simulink model "WEankle_controllerMaarten_2018"  (R2018b)
settings: Solver=FixedStepDiscrete  StartTime=0.0  StopTime=inf  FixedStep=sampleTime  RelTol=1e-3
PreLoadFcn:
  | init
undefined symbols (not defined in the file or in its folder): DiscIntNeverNeededParam, forceplate, Joint_params, sampleTime
libraries: simulink x21, WE2_library x9, dspsigops x6, dspfdesign x3
(part 2 of 4)

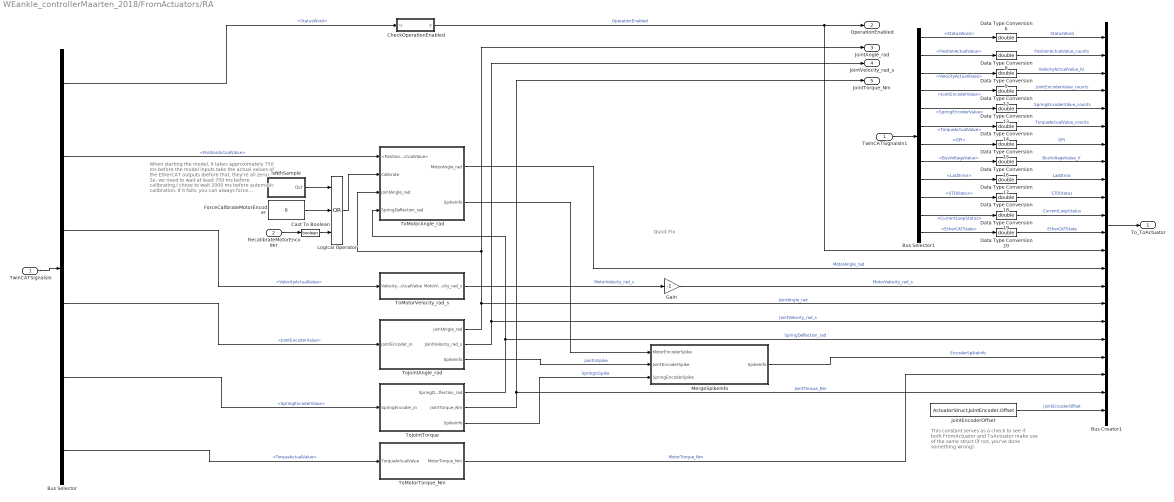
== system WEankle_controllerMaarten_2018/FromActuators/RA ==
  note: Quick Fix
  note: When starting the model, it takes approximately 750 ms before the model inputs take the actual values of the EtherCAT outputs (before that, they're all zero). So, we need to wait at least 750 ms before calibrating.I chose to wait 2000 ms before automatic calibration.
      |
      | If it fails, you can always force re-calibration.
  note: This constant serves as a check to see if both FromActuator and ToActuator make use of the same struct (if not, you've done something wrong).
  TwinCATSignalsIn : Inport  OutDataTypeStr=Bus: WE_InputBus
  RecalibrateMotorEncoder : Inport  Port=2
  Bus Creator1 : BusCreator  Inputs=22  OutDataTypeStr=Bus: WE_ToToActuatorBus  NonVirtualBus=on
      settings: InheritFromInputs=off
  Bus Selector : BusSelector  OutputSignals=StatusWord,PositionActualValue,VelocityActualValue,JointEncoderValue,SpringEncoderValue,TorqueActualValue
  Bus Selector1 : BusSelector  OutputSignals=StatusWord,PositionActualValue,VelocityActualValue,JointEncoderValue,SpringEncoderValue,TorqueActualValue,GPI,BusVoltageValue,LastError,STOStatus,CurrentLoopStatus,EtherCATState
  Cast To Boolean : DataTypeConversion  OutDataTypeStr=boolean
  CheckOperationEnabled : MATLAB Function  TreatAsAtomicUnit=on
  Data Type Conversion{6,8..9,12..20} (12 alike) : DataTypeConversion  OutDataTypeStr=double
  ForceCalibrateMotorEncoder : Constant  Value=0
      settings: OpenFcn=set_param(gcb,'Value','1');tname = ['toggletimer_' gcb];delete(timerfind('name',tname));t = timer('timerfcn', ['set_param(''',gcb,''',''Value'',''0'')'],'executionmode','singleshot','startdelay',1,'name',tname);start(t);
      mask Display: fprintf('PushToTrigger\n%s',get_param(gcb,'value'))
  Gain : Gain  Gain=-1
  IsNthSample : Subsystem  InitFcn=|  mask{N=2000}
      | return; %Disable this becasue it doesnt work!                                                                                                                                                          
      | h = gcb;                                                                                                                                                                                               
      | n = 0; % Number of enable blocks detected upstream                                                                                                                                                     
      | t = []; % type of enable blocks                                                                                                                                                                        
      | while 1,                                                                                                                                                                                               
      |   % Find parent                                                                                                                                                                                        
      |   h = get_param(h,'parent');                                                                                                                                                                           
      |   if (strcmp(h,'')),                                                                                                                                                                                   
      |       % Then we've reached the root                                                                                                                                                                    
      |       break;                                                                                                                                                                                           
      |   end;                                                                                                                                                                                                 
      |   % and check if it has an enable port                                                                                                                                                                 
      |   e = find_system(h,'searchdepth',1, 'BlockType','EnablePort');                                                                                                                                        
      |   if (numel(e)==1),                                                                                                                                                                                    
      |     s = get_param(e{1},'StatesWhenEnabling');                                                                                                                                                          
      |     n=n+1;                                                                                                                                                                                             
      |     if (strcmp(s,'held')),                                                                                                                                                                             
      |         t=[t;'h']; %#ok<AGROW>                                                                                                                                                                         
      |     else                                                                                                                                                                                               
      |         t=[t;'r']; %#ok<AGROW>                                                                                                                                                                         
      |     end;                                                                                                                                                                                               
      |   elseif (numel(e)>1),                                                                                                                                                                                 
      |       error('hun? Multiple enable blocks!')                                                                                                                                                            
      |   end;                                                                                                                                                                                                 
      | end;                                                                                                                                                                                                   
      |                                                                                                                                                                                                        
      | if (n==0),                                                                                                                                                                                             
      |     warning('Warning: %s - The block is not inside an enabled block',gcb)                                                                                                                              
      | elseif (n==1),                                                                                                                                                                                         
      |     if (t(1)=='r')                                                                                                                                                                                     
      |         % This is okay, do nothing                                                                                                                                                                     
      |     else                                                                                                                                                                                               
      |         warning('Warning: %s - This block is inside an enabled block which has its "State when enabling" set to "held". Usually you want it set to "reset" for correct operation.',gcb);               
      |     end;                                                                                                                                                                                               
      | else % n>1                                                                                                                                                                                             
      |     warning('Warning: %s - This block is inside multiple nested enabled blocks. Check which blocks are "held" and which are "reset". You usually want to have at least one "reset" enabled block',gcb);
      | end;
  JointEncoderOffset : Constant  Value=ActuatorStruct.JointEncoder.Offset
  Logical Operator : Logic  Operator=OR  Inputs=3  AllPortsSameDT=off  OutDataTypeStr=boolean
  MergeSpikeInfo : Subsystem
  ToJointAngle_rad : Subsystem
  ToJointTorque : Subsystem
  ToMotorAngle_rad : Subsystem
  ToMotorTorque_Nm : Subsystem
  ToMotorVelocity_rad_s : Subsystem
  TwinCATSignalsIn1 : InportShadow  OutDataTypeStr=Bus: WE_InputBus
  To_ToActuator : Outport  OutDataTypeStr=Bus: WE_ToToActuatorBus  VectorParamsAs1DForOutWhenUnconnected=off
  OperationEnabled : Outport  Port=2  VectorParamsAs1DForOutWhenUnconnected=off
  JointAngle_rad : Outport  Port=3  VectorParamsAs1DForOutWhenUnconnected=off
  JointVelocity_rad_s : Outport  Port=4  VectorParamsAs1DForOutWhenUnconnected=off
  JointTorque_Nm : Outport  Port=5  VectorParamsAs1DForOutWhenUnconnected=off
  wires:
  Cast To Boolean/1 -> Logical Operator/3
  ToMotorAngle_rad/1(MotorAngle_rad) -> Bus Creator1/14  "MotorAngle_rad"
  Logical Operator/1 -> ToMotorAngle_rad/2(Calibrate)
  Bus Selector/2 -> ToMotorAngle_rad/1(<PositionActualValue>)  "<PositionActualValue>"
  ToMotorAngle_rad/2(SpikeInfo) -> MergeSpikeInfo/1(MotorEncoderSpike)
  MergeSpikeInfo/1(SpikeInfo) -> Bus Creator1/19  "EncoderSpikeInfo"
  Bus Selector1/12 -> Data Type Conversion20/1  "<EtherCATState>"
  Bus Selector1/11 -> Data Type Conversion19/1  "<CurrentLoopStatus>"
  Bus Selector1/10 -> Data Type Conversion18/1  "<STOStatus>"
  Bus Selector1/9 -> Data Type Conversion17/1  "<LastError>"
  Bus Selector1/8 -> Data Type Conversion16/1  "<BusVoltageValue>"
  Bus Selector1/7 -> Data Type Conversion15/1  "<GPI>"
  Bus Selector1/6 -> Data Type Conversion14/1  "<TorqueActualValue>"
  Bus Selector1/5 -> Data Type Conversion13/1  "<SpringEncoderValue>"
  Bus Selector1/4 -> Data Type Conversion12/1  "<JointEncoderValue>"
  Bus Selector1/3 -> Data Type Conversion9/1  "<VelocityActualValue>"
  Bus Selector1/2 -> Data Type Conversion8/1  "<PositionActualValue>"
  Data Type Conversion20/1 -> Bus Creator1/12  "EtherCATState"
  Data Type Conversion19/1 -> Bus Creator1/11  "CurrentLoopStatus"
  Data Type Conversion18/1 -> Bus Creator1/10  "STOStatus"
  Data Type Conversion17/1 -> Bus Creator1/9  "LastError"
  Data Type Conversion16/1 -> Bus Creator1/8  "BusVoltageValue_V"
  Data Type Conversion15/1 -> Bus Creator1/7  "GPI"
  Data Type Conversion14/1 -> Bus Creator1/6  "TorqueActualValue_counts"
  Data Type Conversion13/1 -> Bus Creator1/5  "SpringEncoderValue_counts"
  Data Type Conversion12/1 -> Bus Creator1/4  "JointEncoderValue_counts"
  Data Type Conversion9/1 -> Bus Creator1/3  "VelocityActualValue_IU"
  Data Type Conversion8/1 -> Bus Creator1/2  "PositionActualValue_counts"
  Data Type Conversion6/1 -> Bus Creator1/1  "StatusWord"
  Bus Selector1/1 -> Data Type Conversion6/1  "<StatusWord>"
  TwinCATSignalsIn1/1 -> Bus Selector1/1
  Bus Selector/6 -> ToMotorTorque_Nm/1(TorqueActualValue)  "<TorqueActualValue>"
  Bus Selector/5 -> ToJointTorque/1(SpringEncoder_in)  "<SpringEncoderValue>"
  Bus Selector/4 -> ToJointAngle_rad/1(JointEncoder_in)  "<JointEncoderValue>"
  RecalibrateMotorEncoder/1 -> Cast To Boolean/1
  ToMotorVelocity_rad_s/1(MotorVelocity_rad_s) -> Gain/1  "MotorVelocity_rad_s"
  ToMotorTorque_Nm/1(MotorTorque_Nm) -> Bus Creator1/20  "MotorTorque_Nm"
  ToJointTorque/3(SpikeInfo) -> MergeSpikeInfo/3(SpringEncoderSpike)  "SpringIsSpike"
  ToJointAngle_rad/3(SpikeInfo) -> MergeSpikeInfo/2(JointEncoderSpike)  "JointIsSpike"
  JointEncoderOffset/1 -> Bus Creator1/22  "JointEncoderOffset"
  Bus Creator1/1 -> To_ToActuator/1
  CheckOperationEnabled/1(y) -> OperationEnabled/1, Bus Creator1/13  "OperationEnabled"
  ToJointTorque/2(JointTorque_Nm) -> Bus Creator1/21, JointTorque_Nm/1  "JointTorque_Nm"
  ToJointAngle_rad/2(JointVelocity_rad_s) -> Bus Creator1/17, JointVelocity_rad_s/1  "JointVelocity_rad_s"
  ToJointAngle_rad/1(JointAngle_rad) -> ToMotorAngle_rad/3(JointAngle_rad), JointAngle_rad/1, Bus Creator1/16  "JointAngle_rad"
  ToJointTorque/1(SpringDeflection_rad) -> ToMotorAngle_rad/4(SpringDeflection_rad), Bus Creator1/18  "SpringDeflection_rad"
  IsNthSample/1(Out) -> Logical Operator/1
  ForceCalibrateMotorEncoder/1 -> Logical Operator/2
  TwinCATSignalsIn/1 -> Bus Selector/1
  Bus Selector/1 -> CheckOperationEnabled/1(u)  "<StatusWord>"
  Bus Selector/3 -> ToMotorVelocity_rad_s/1(VelocityActualValue)  "<VelocityActualValue>"
  Gain/1 -> Bus Creator1/15  "MotorVelocity_rad_s"

== system WEankle_controllerMaarten_2018/Ankle Controller/COMverror and perturbation/COMvError ==
  note: This input signal should be taken from original, but the data is not good before the filter because of the Qualisys sample rate
  Signaltime : Inport
  trigger : Inport  Port=2
  xPosCOM : Inport  Port=3
  Constant : Constant  Value=5
  Constant1 : Constant  Value=1.5
  Data lost detection : Subsystem
  MATLAB Function1 : MATLAB Function  TreatAsAtomicUnit=on
  PertDetection : Subsystem
  PerturbationDetectionFromError : MATLAB Function  TreatAsAtomicUnit=on
  Signal learner : Subsystem
  Terminator : Terminator
  Terminator1 : Terminator
  Terminator8 : Terminator
  to mm : Gain  Gain=1000
  PushDetected : Outport  VectorParamsAs1DForOutWhenUnconnected=off
  COMv_meas : Outport  Port=2  VectorParamsAs1DForOutWhenUnconnected=off
  COMv_ref : Outport  Port=3  VectorParamsAs1DForOutWhenUnconnected=off
  COMv_error : Outport  Port=4  VectorParamsAs1DForOutWhenUnconnected=off
  tag scope: DataLost=global, ShutDown=global
  wires:
  to mm/1 -> Signal learner/3(xPosCOM)
  [ShutDown] -> MATLAB Function1/1(ShutDown)
  PertDetection/1(PertDetect) -> MATLAB Function1/2(PertDetect)
  Signal learner/6(ShutDown) -> [ShutDown]
  [DataLost] -> PerturbationDetectionFromError/6(DataLost)
  Data lost detection/2(DataLost) -> [DataLost]  "DataLost"
  Constant1/1 -> PerturbationDetectionFromError/5(threshPert)
  Signal learner/3(Input filtered) -> Data lost detection/1(Input signal), COMv_meas/1  "InputFiltered"
  Data lost detection/1(New error) -> COMv_error/1, PerturbationDetectionFromError/3(signal)  "Error"
  Signal learner/4(learned) -> COMv_ref/1  "SignalLearned"
  MATLAB Function1/1(TriggerPush) -> PushDetected/1
  Data lost detection/3(avoid) -> PertDetection/3(avoid)
  Signal learner/5(Perturbation detected FromInput) -> PertDetection/2(PertFromInputSignal)
  PerturbationDetectionFromError/1(push) -> PertDetection/1(PertFromError)  "PertFromError"
  Constant/1 -> PerturbationDetectionFromError/4(n_rep)
  Signal learner/2(error) -> Data lost detection/2(ErrorIn)
  xPosCOM/1 -> to mm/1
  Signaltime/1 -> PerturbationDetectionFromError/1(t), Signal learner/1(Signaltime)
  trigger/1 -> Signal learner/2(trigger), PerturbationDetectionFromError/2(trigger)  "trigger"
  PerturbationDetectionFromError/2(maxAver) -> Terminator8/1
  PerturbationDetectionFromError/3(rangeAver) -> Terminator1/1
  Signal learner/1(original) -> Terminator/1

== system WEankle_controllerMaarten_2018/Ankle Controller/COMverror and perturbation/TriggerPerturbation ==
  note: Put it in 4
  note: I have to try the pull perturbation in the pusher and its response
      | and change the amplitude based on that
  note: 1 - only push
      | 0 - push and pull
  In1 : Inport
  In2 : Inport  Port=2
  SingleR : Inport  Port=3
  SingleL : Inport  Port=4
  In5 : Inport  Port=5
  In6 : Inport  Port=6
  Delay : Delay  DelayLength=200
  Demux2 : Demux  Outputs=2
  GainP : Gain  Gain=4
  MATLAB Function2 : MATLAB Function  TreatAsAtomicUnit=on
  Multiply1 : Product
  Perturbation sync gait phase1 : Subsystem
  PushOrPull : MATLAB Function  TreatAsAtomicUnit=on
  Selector4 : Selector  InputPortWidth=6  IndexOptions=Index vector (dialog)  Indices=3  OutputSizes=1
  Switch2 : Switch  Criteria=u2 > Threshold
  Terminator1 : Terminator
  Type of perturbations (random) : Constant  Value=[1 1 1 1 1 1 1 1 1]
  VectorOnlyPush : Constant
  VectorPushPull : Constant  Value=[1 -1 1 1 1 -1 -1 1 -1 -1 1 -1]
  PerturbationTrigger : Outport
  wires:
  In2/1 -> Switch2/2
  In1/1 -> Multiply1/1
  SingleR/1 -> MATLAB Function2/1(SingleR)
  In5/1 -> Demux2/1
  SingleL/1 -> MATLAB Function2/2(SingleL)
  Delay/1 -> PushOrPull/3(Delivered)
  PushOrPull/1(NewPert) -> GainP/1  "New pert"
  Perturbation sync gait phase1/3(allow) -> Terminator1/1
  Selector4/1 -> MATLAB Function2/5(GRFzL)
  VectorOnlyPush/1 -> Switch2/1
  Type of perturbations (random)/1 -> MATLAB Function2/6(TypePert)
  MATLAB Function2/1(Trigger) -> Perturbation sync gait phase1/1(trigger)  "trigger"
  Switch2/1 -> PushOrPull/2(vectorPushPull)  "vectorPert"
  Demux2/1 -> MATLAB Function2/3(PhaseL)  "PhaseL"
  VectorPushPull/1 -> Switch2/3
  In6/1 -> Selector4/1
  Demux2/2 -> MATLAB Function2/4(PhaseR)  "PhaseR"
  GainP/1 -> Multiply1/2
  Perturbation sync gait phase1/1(Pert sync) -> PushOrPull/1(Perturb)  "pert"
  Multiply1/1 -> PerturbationTrigger/1
  Perturbation sync gait phase1/2(Delivered) -> MATLAB Function2/7(Delivered), Delay/1  "Delivered"

== system WEankle_controllerMaarten_2018/Ankle Controller/Gait Phase detection/COP detection (treadmill) ==
  note: Detection of ground contact when wearing exo 200 (without exo 80)
  note: Number coding :
      | 1 = LIFOR
      | 2 = SSL
      | 3 = RIFOL
      | 4 = SSR
  note: NOTE 1
      | This block of course assumes that the left leg stays on the left belt, and the right one on the right belt.
  note: y-forward
      | x-lateral
      | z-up
  Left GRF : Inport
  Right GRF : Inport  Port=2
  Constant1 : Constant  Value=2*pi*50
  Constant2 : Constant  Value=200
  Constant3 : Constant  Value=0.001
  Gain1 : Gain
  Gain2 : Gain
  Get_COPL : Subsystem  TreatAsAtomicUnit=on
  Get_COPR : Subsystem  TreatAsAtomicUnit=on
  LEFT Fz : Selector  InputPortWidth=6  IndexOptions=Index vector (dialog)  Indices=[3]  OutputSizes=1
  MATLAB Function1 : MATLAB Function  TreatAsAtomicUnit=on
  MATLAB Function2 : MATLAB Function  TreatAsAtomicUnit=on
  RIGHT Fz : Selector  InputPortWidth=6  IndexOptions=Index vector (dialog)  Indices=[3]  OutputSizes=1
  Relational Operator : RelationalOperator  OutDataTypeStr=boolean  RndMeth=Simplest
  Relational Operator1 : RelationalOperator  OutDataTypeStr=boolean  RndMeth=Simplest
  COPLxy : Outport  VectorParamsAs1DForOutWhenUnconnected=off
  COPRxy : Outport  Port=2  VectorParamsAs1DForOutWhenUnconnected=off
  wires:
  MATLAB Function2/1(y) -> Get_COPR/1(grf), RIGHT Fz/1
  RIGHT Fz/1 -> Gain1/1
  LEFT Fz/1 -> Gain2/1
  Relational Operator/1 -> Get_COPL/Enable
  Relational Operator1/1 -> Get_COPR/Enable
  Constant1/1 -> MATLAB Function1/2(OmegaFilter), MATLAB Function2/2(OmegaFilter)
  MATLAB Function1/1(y) -> Get_COPL/1(grf), LEFT Fz/1
  Gain2/1 -> Relational Operator/1
  Gain1/1 -> Relational Operator1/1
  Left GRF/1 -> MATLAB Function1/1(x)
  Right GRF/1 -> MATLAB Function2/1(x)
  Constant2/1 -> Relational Operator/2, Relational Operator1/2
  Get_COPL/1(COPL) -> COPLxy/1
  Get_COPR/1(COPR) -> COPRxy/1
  Constant3/1 -> MATLAB Function1/3(sampleTime), MATLAB Function2/3(sampleTime)

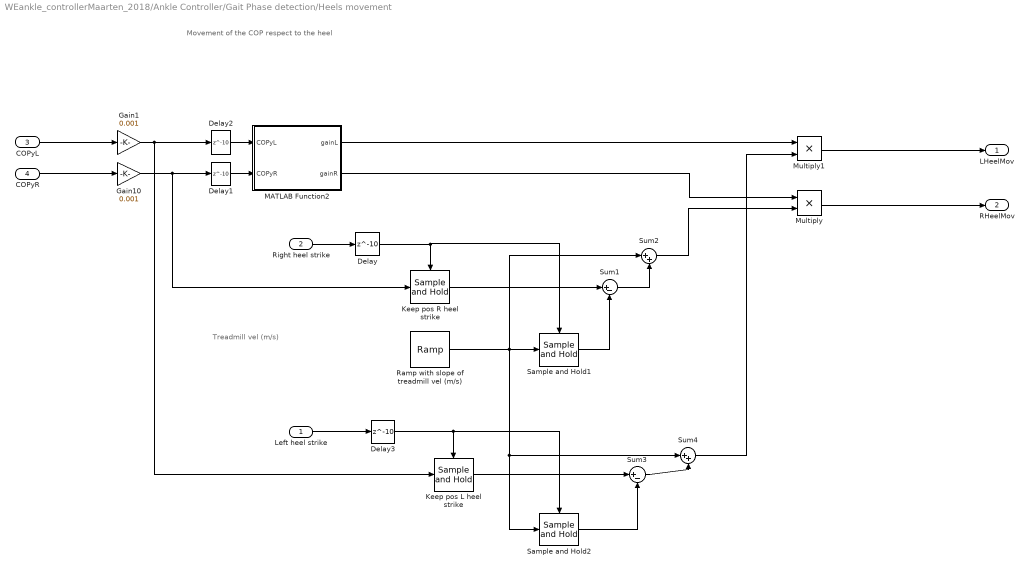
== system WEankle_controllerMaarten_2018/Ankle Controller/Gait Phase detection/Heels movement ==
  note: Movement of the COP respect to the heel
  note: Treadmill vel (m/s)
  Left heel strike : Inport
  Right heel strike : Inport  Port=2
  COPyL : Inport  Port=3
  COPyR : Inport  Port=4
  Delay{,1..3} (4 alike) : Delay  DelayLength=10
  Gain1 : Gain  Gain=0.001
  Gain10 : Gain  Gain=0.001
  Keep pos L heel strike : dspsigops/Sample and Hold  trig=Rising edge  initCond=0  latchinput=off
  Keep pos R heel strike : dspsigops/Sample and Hold  trig=Rising edge  initCond=0  latchinput=off
  MATLAB Function2 : MATLAB Function  TreatAsAtomicUnit=on
  Multiply : Product
  Multiply1 : Product
  Ramp with slope of treadmill vel (m/s) : simulink/Sources/Ramp  slope=-0.56  start=0  InitialOutput=0
  Sample and Hold1 : dspsigops/Sample and Hold  trig=Rising edge  initCond=0  latchinput=off
  Sample and Hold2 : dspsigops/Sample and Hold  trig=Rising edge  initCond=0  latchinput=off
  Sum1 : Sum  Inputs=|+-
  Sum2 : Sum  Inputs=|++
  Sum3 : Sum  Inputs=|+-
  Sum4 : Sum  Inputs=|++
  LHeelMov : Outport  VectorParamsAs1DForOutWhenUnconnected=off
  RHeelMov : Outport  Port=2  VectorParamsAs1DForOutWhenUnconnected=off
  wires:
  Sum2/1 -> Multiply/2
  Delay1/1 -> MATLAB Function2/2(COPyR)
  Ramp with slope of treadmill vel (m/s)/1 -> Sum4/1, Sample and Hold2/1, Sum2/1, Sample and Hold1/1
  Multiply/1 -> RHeelMov/1
  MATLAB Function2/2(gainR) -> Multiply/1
  Keep pos R heel strike/1 -> Sum1/1
  COPyR/1 -> Gain10/1
  Delay/1 -> Keep pos R heel strike/Trigger, Sample and Hold1/Trigger
  Gain10/1 -> Keep pos R heel strike/1, Delay1/1
  Sample and Hold1/1 -> Sum1/2
  Sum1/1 -> Sum2/2
  Right heel strike/1 -> Delay/1
  Delay2/1 -> MATLAB Function2/1(COPyL)
  Gain1/1 -> Delay2/1, Keep pos L heel strike/1
  COPyL/1 -> Gain1/1
  MATLAB Function2/1(gainL) -> Multiply1/1
  Left heel strike/1 -> Delay3/1
  Delay3/1 -> Sample and Hold2/Trigger, Keep pos L heel strike/Trigger
  Keep pos L heel strike/1 -> Sum3/1
  Sample and Hold2/1 -> Sum3/2
  Sum3/1 -> Sum4/2
  Sum4/1 -> Multiply1/2
  Multiply1/1 -> LHeelMov/1

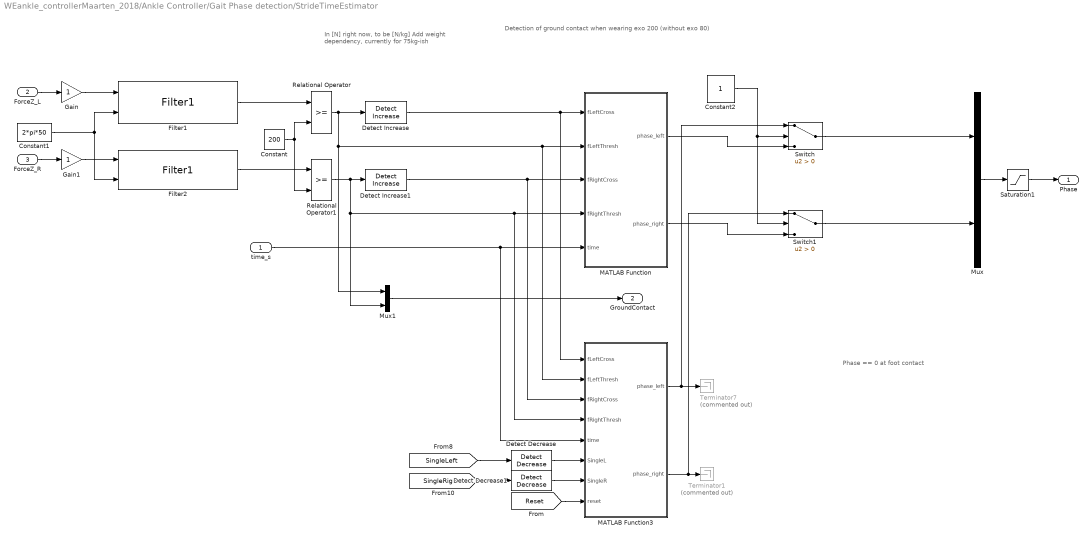
== system WEankle_controllerMaarten_2018/Ankle Controller/Gait Phase detection/StrideTimeEstimator ==
  note: In [N] right now, to be [N/kg]
      | Add weight dependency, currently for 75kg-ish
  note: Detection of ground contact when wearing exo 200 (without exo 80)
  note: Phase == 0 at foot contact
  time_s : Inport
  ForceZ_L : Inport  Port=2
  ForceZ_R : Inport  Port=3
  Constant : Constant  Value=200
  Constant1 : Constant  Value=2*pi*50
  Constant2 : Constant  VectorParams1D=off  SampleTime=-1
  Detect Decrease : simulink/Logic and Bit Operations/Detect Decrease  vinit=0.0  OutDataTypeStr=boolean
  Detect Decrease1 : simulink/Logic and Bit Operations/Detect Decrease  vinit=0.0  OutDataTypeStr=boolean
  Detect Increase : simulink/Logic and Bit Operations/Detect Increase  vinit=0.0  OutDataTypeStr=boolean
  Detect Increase1 : simulink/Logic and Bit Operations/Detect Increase  vinit=0.0  OutDataTypeStr=boolean
  Filter1 : WE2_library/FromActuator/ToGearboxAngle_rad/FilterFourthOrder/Filter1  sampleTime=sampleTime
  Filter2 : WE2_library/FromActuator/ToGearboxAngle_rad/FilterFourthOrder/Filter1  sampleTime=sampleTime
  Gain : Gain
  Gain1 : Gain
  MATLAB Function : MATLAB Function  TreatAsAtomicUnit=on
  MATLAB Function3 : MATLAB Function  TreatAsAtomicUnit=on
  Mux : Mux  Inputs=2
  Mux1 : Mux  Inputs=2
  Relational Operator : RelationalOperator  OutDataTypeStr=boolean  RndMeth=Simplest
  Relational Operator1 : RelationalOperator  OutDataTypeStr=boolean  RndMeth=Simplest
  Saturation1 : Saturate  UpperLimit=100  LowerLimit=0
  Switch : Switch  Criteria=u2 > Threshold
  Switch1 : Switch  Criteria=u2 > Threshold
  Terminator1 : Terminator  Commented=on
  Terminator7 : Terminator  Commented=on
  Phase : Outport  VectorParamsAs1DForOutWhenUnconnected=off
  GroundContact : Outport  Port=2  VectorParamsAs1DForOutWhenUnconnected=off
  wires:
  Gain1/1 -> Filter2/1
  Gain/1 -> Filter1/1
  Constant1/1 -> Filter1/2, Filter2/2
  Filter1/1 -> Relational Operator/1
  Filter2/1 -> Relational Operator1/1
  Mux1/1 -> GroundContact/1
  Mux/1 -> Saturation1/1
  Saturation1/1 -> Phase/1
  Switch/1 -> Mux/1
  Detect Increase1/1 -> MATLAB Function3/3(fRightCross), MATLAB Function/3(fRightCross)
  Detect Increase/1 -> MATLAB Function3/1(fLeftCross), MATLAB Function/1(fLeftCross)
  Relational Operator1/1 -> Detect Increase1/1, MATLAB Function3/4(fRightThresh), MATLAB Function/4(fRightThresh), Mux1/2
  Relational Operator/1 -> Detect Increase/1, MATLAB Function3/2(fLeftThresh), MATLAB Function/2(fLeftThresh), Mux1/1
  Constant/1 -> Relational Operator1/2, Relational Operator/2
  time_s/1 -> MATLAB Function3/5(time), MATLAB Function/5(time)
  ForceZ_R/1 -> Gain1/1
  ForceZ_L/1 -> Gain/1
  Detect Decrease/1 -> MATLAB Function3/6(SingleL)
  Detect Decrease1/1 -> MATLAB Function3/7(SingleR)
  [SingleRight] -> Detect Decrease1/1
  [SingleLeft] -> Detect Decrease/1
  MATLAB Function3/1(phase_left) -> Switch/1, Terminator7/1
  MATLAB Function3/2(phase_right) -> Switch1/1, Terminator1/1
  Switch1/1 -> Mux/2
  MATLAB Function/2(phase_right) -> Switch1/3
  MATLAB Function/1(phase_left) -> Switch/3
  Constant2/1 -> Switch1/2, Switch/2
  [Reset] -> MATLAB Function3/8(reset)

== system WEankle_controllerMaarten_2018/Ankle Controller/Gait Phase detection/Subsystem ==
  In1 : Inport
  Constant : Constant  Value=5
  Delay2 : Delay  DelayLength=1
  Lowpass Filter2 : dspfdesign/Lowpass Filter  FilterType=IIR  DesignForMinimumOrder=on  FilterOrder=50  PassbandFrequency=40  StopbandFrequency=50  PassbandRipple=0.1  StopbandAttenuation=40  InheritSampleRate=off  SampleRate=1000  SimulateUsing=Interpreted execution  roundingMode=Floor  coeffsDataTypeStr=fixdt(1,16)
  MATLAB Function : MATLAB Function  TreatAsAtomicUnit=on
  Rate Transition : RateTransition
  Out1 : Outport  VectorParamsAs1DForOutWhenUnconnected=off
  wires:
  MATLAB Function/1(y) -> Out1/1
  Rate Transition/1 -> Lowpass Filter2/1
  Constant/1 -> MATLAB Function/4(th)
  Lowpass Filter2/1 -> MATLAB Function/1(f)  "prev"
  Delay2/1 -> MATLAB Function/3(nf_1)
  In1/1 -> Delay2/1, MATLAB Function/2(nf), Rate Transition/1

== system WEankle_controllerMaarten_2018/Ankle Controller/Gait Phase detection/Subsystem1 ==
  In1 : Inport
  Constant : Constant  Value=5
  Delay2 : Delay  DelayLength=1
  Lowpass Filter2 : dspfdesign/Lowpass Filter  FilterType=IIR  DesignForMinimumOrder=on  FilterOrder=50  PassbandFrequency=40  StopbandFrequency=50  PassbandRipple=0.1  StopbandAttenuation=40  InheritSampleRate=off  SampleRate=1000  SimulateUsing=Interpreted execution  roundingMode=Floor  coeffsDataTypeStr=fixdt(1,16)
  MATLAB Function : MATLAB Function  TreatAsAtomicUnit=on
  Rate Transition : RateTransition
  Out1 : Outport  VectorParamsAs1DForOutWhenUnconnected=off
  wires:
  MATLAB Function/1(y) -> Out1/1
  Rate Transition/1 -> Lowpass Filter2/1
  Constant/1 -> MATLAB Function/4(th)
  Lowpass Filter2/1 -> MATLAB Function/1(f)  "prev"
  Delay2/1 -> MATLAB Function/3(nf_1)
  In1/1 -> Delay2/1, MATLAB Function/2(nf), Rate Transition/1

== system WEankle_controllerMaarten_2018/FromActuators/RA/IsNthSample ==
  note: This block outputs 1 on the Nth sample of the enabled block,
      | zero otherwise. Note that this is 0-based (e.g., N=3 is the fourth
      | sample). Note that it only works if the enable port has
      | "States when enabled" set to "reset"!
  Counter Free-Running : simulink/Sources/Counter Free-Running  NumBits=32  tsamp=-1
  N : Constant  Value=N
  Relational Operator : RelationalOperator  Operator===  OutDataTypeStr=boolean  RndMeth=Nearest
  Out : Outport  VectorParamsAs1DForOutWhenUnconnected=off
  wires:
  Relational Operator/1 -> Out/1
  Counter Free-Running/1 -> Relational Operator/1
  N/1 -> Relational Operator/2

== system WEankle_controllerMaarten_2018/FromActuators/RA/MergeSpikeInfo ==
  note: This element contains all spikeinfo bits of all encoders:
      |
      | Bits:
      | 31-12: -
      | 11: -
      | 10: MotorEasfencoderIsExtrapolated
      |  9: MotorEncoderIsRepeatedValue
      |  8: MotorEncoderIsSpike
      |  7: -
      |  6: JointEncoderIsExtrapolated
      |  5: JointEasfencoderIsRepeatedValue
      |  4: JointEncoderIsSpike
      |  3: -
      |  2: SpringEncoderIsExtrapolated
      |  1: SpringasfederIsRepeatedValue
      |  0: SpringEncoderIsSpike
  MotorEncoderSpike : Inport
  JointEncoderSpike : Inport  Port=2
  SpringEncoderSpike : Inport  Port=3
  Add : Sum  Inputs=+++
  Gain1 : Gain  Gain=2^4
  Gain2 : Gain  Gain=2^8
  SpikeInfo : Outport  VectorParamsAs1DForOutWhenUnconnected=off
  wires:
  Gain2/1 -> Add/1
  Gain1/1 -> Add/2
  MotorEncoderSpike/1 -> Gain2/1
  JointEncoderSpike/1 -> Gain1/1
  SpringEncoderSpike/1 -> Add/3
  Add/1 -> SpikeInfo/1

== system WEankle_controllerMaarten_2018/FromActuators/RA/ToJointAngle_rad ==
  note: Normally, this should be zero, but in rare cases you can tweak the system with this.
  note: bit 2: OutputValue IsExtrapolated
      | bit 1: IsRepeatedValue
      | bit 0: IsSpike
  JointEncoder_in : Inport
  Constant : Constant  Value=2*pi
  Data Type Conversion : DataTypeConversion  OutDataTypeStr=double
  Data Type Conversion1 : DataTypeConversion  OutDataTypeStr=double
  FilterFourthOrder : Subsystem
  JointEncoderCountsPerRev : Constant  Value=ActuatorStruct.JointEncoder.Counts_rev
  JointEncoderOffset : Constant  Value=ActuatorStruct.JointEncoder.Offset
  JointEncoderOffset2 : Constant  Value=ActuatorStruct.JointEncoder.Counts_rev
  MATLAB Function : MATLAB Function  TreatAsAtomicUnit=on
  MATLAB Function1 : MATLAB Function  TreatAsAtomicUnit=on
  ManualOffset : Constant  Value=0
  Omega1 : Constant  Value=2*pi*100  OutDataTypeStr=double
  Product : Product  Inputs=*/*
  RomIncludesZero : Constant  Value=ActuatorStruct.JointEncoder.ROMIncludesZero
  SpikeAndRepeatFilter : Subsystem
  SpikeFilterWindowGrowthRate : Constant  Value=ActuatorStruct.JointEncoder.SpikeFilter.WindowGrowthRate_rad_sample
  Subtract : Sum  Inputs=+--
  TakeDerivative : Subsystem
  JointAngle_rad : Outport  VectorParamsAs1DForOutWhenUnconnected=off
  JointVelocity_rad_s : Outport  Port=2  VectorParamsAs1DForOutWhenUnconnected=off
  SpikeInfo : Outport  Port=3  VectorParamsAs1DForOutWhenUnconnected=off
  wires:
  SpikeFilterWindowGrowthRate/1 -> SpikeAndRepeatFilter/2(SpikeWindowGrowthRate)
  SpikeAndRepeatFilter/2(SpikeInfo) -> SpikeInfo/1
  Data Type Conversion1/1 -> Subtract/2
  MATLAB Function1/1(y) -> Data Type Conversion1/1
  RomIncludesZero/1 -> MATLAB Function/3(dowrap), MATLAB Function1/3(dowrap)
  JointEncoderOffset2/1 -> MATLAB Function/2(counts_rev), MATLAB Function1/2(counts_rev)
  MATLAB Function/1(y) -> Data Type Conversion/1
  Data Type Conversion/1 -> Subtract/1
  Product/1 -> SpikeAndRepeatFilter/1(In)
  ManualOffset/1 -> Subtract/3
  JointEncoderCountsPerRev/1 -> Product/2
  Subtract/1 -> Product/1
  Constant/1 -> Product/3
  JointEncoder_in/1 -> MATLAB Function/1(u)
  FilterFourthOrder/1(Out) -> JointVelocity_rad_s/1
  SpikeAndRepeatFilter/1(Out) -> JointAngle_rad/1, TakeDerivative/1(In1)
  Omega1/1 -> FilterFourthOrder/2(Omega)
  JointEncoderOffset/1 -> MATLAB Function1/1(u)
  TakeDerivative/1(Out1) -> FilterFourthOrder/1(In)

== system WEankle_controllerMaarten_2018/FromActuators/RA/ToJointTorque ==
  note: bit 2: OutputValue IsExtrapolated
      | bit 1: IsRepeatedValue
      | bit 0: IsSpike
  note: Normally, this should be zero, but in rarecases you can tweak the system with this.
  SpringEncoder_in : Inport
  Constant : Constant  Value=2*pi
  Data Type Conversion : DataTypeConversion  OutDataTypeStr=double
  EncoderOffset_counts : Display
  JointEncoderOffset2 : Constant  Value=ActuatorStruct.SpringEncoder.Counts_rev
  MATLAB Function : MATLAB Function  TreatAsAtomicUnit=on
  MATLAB Function1 : MATLAB Function  TreatAsAtomicUnit=on
  ManualOffset : Constant  Value=100
  Product : Product  Inputs=*/*
  Product2 : Product  Inputs=**
  RomIncludesZero : Constant  Value=ActuatorStruct.SpringEncoder.ROMIncludesZero
  SpikeAndRepeatFilter : WE2_library/FromActuator/ToJointAngle_rad/SpikeAndRepeatFilter  SystemSampleTime=-1
  SpikeFilterWindowGrowthRate : Constant  Value=ActuatorStruct.SpringEncoder.SpikeFilter.WindowGrowthRate_rad_sample
  SpringEncoderCountsPerRev : Constant  Value=ActuatorStruct.SpringEncoder.Counts_rev
  SpringEncoderOffset : Constant  Value=ActuatorStruct.SpringEncoder.Offset
  SpringStiffness : Constant  Value=ActuatorStruct.SpringStiffness_Nm_rad
  Subtract : Sum  Inputs=+--
  SpringDeflection_rad : Outport  VectorParamsAs1DForOutWhenUnconnected=off
  JointTorque_Nm : Outport  Port=2  VectorParamsAs1DForOutWhenUnconnected=off
  SpikeInfo : Outport  Port=3  VectorParamsAs1DForOutWhenUnconnected=off
  wires:
  SpikeFilterWindowGrowthRate/1 -> SpikeAndRepeatFilter/2
  SpikeAndRepeatFilter/1 -> SpringDeflection_rad/1, Product2/2
  Product/1 -> SpikeAndRepeatFilter/1
  SpikeAndRepeatFilter/2 -> SpikeInfo/1
  Product2/1 -> JointTorque_Nm/1
  MATLAB Function1/1(y) -> Subtract/2
  MATLAB Function/1(y) -> Data Type Conversion/1
  RomIncludesZero/1 -> MATLAB Function/3(dowrap), MATLAB Function1/3(dowrap)
  JointEncoderOffset2/1 -> MATLAB Function/2(counts_rev), MATLAB Function1/2(counts_rev)
  SpringEncoder_in/1 -> MATLAB Function/1(u)
  Data Type Conversion/1 -> Subtract/1
  SpringStiffness/1 -> Product2/1
  SpringEncoderOffset/1 -> MATLAB Function1/1(u)
  Constant/1 -> Product/3
  Subtract/1 -> EncoderOffset_counts/1, Product/1
  SpringEncoderCountsPerRev/1 -> Product/2
  ManualOffset/1 -> Subtract/3

== system WEankle_controllerMaarten_2018/FromActuators/RA/ToMotorAngle_rad ==
  <PositionActualValue> : Inport
  Calibrate : Inport  Port=2
  JointAngle_rad : Inport  Port=3
  SpringDeflection_rad : Inport  Port=4
  MotorAngle : MATLAB Function  TreatAsAtomicUnit=on  mask{gearboxRatio=ActuatorStruct.GearboxRatio, encoderCounts_rev=ActuatorStruct.MotorEncoder.Counts_rev}
      mask prompts: gearboxRatio "Gearbox Ratio (e.g., -100)"; encoderCounts_rev "Encoder increments per revolution (e.g., 8192)"
  SpikeAndRepeatFilter : WE2_library/FromActuator/ToJointAngle_rad/SpikeAndRepeatFilter  SystemSampleTime=-1
  SpikeFilterWindowGrowthRate : Constant  Value=ActuatorStruct.MotorEncoder.SpikeFilter.WindowGrowthRate_rad_sample
  MotorAngle_rad : Outport  VectorParamsAs1DForOutWhenUnconnected=off
  SpikeInfo : Outport  Port=2  VectorParamsAs1DForOutWhenUnconnected=off
  wires:
  SpikeFilterWindowGrowthRate/1 -> SpikeAndRepeatFilter/2
  SpikeAndRepeatFilter/2 -> SpikeInfo/1
  MotorAngle/1(pos_mot_rad) -> SpikeAndRepeatFilter/1  "MotorAngle_rad"
  SpikeAndRepeatFilter/1 -> MotorAngle_rad/1  "MotorAngle_rad"
  <PositionActualValue>/1 -> MotorAngle/1(pos)
  SpringDeflection_rad/1 -> MotorAngle/3(SpringDeflection_rad)
  JointAngle_rad/1 -> MotorAngle/2(JointAngle_rad)
  Calibrate/1 -> MotorAngle/4(Calibrate)

== system WEankle_controllerMaarten_2018/FromActuators/RA/ToMotorTorque_Nm ==
  note: This block calculates the torque that the motor delivers (or, the current), converted to torque on the output shaft.
  note: Torque_Nm_AfterGearbox = Torque_Nm_Motor * GearboxRatio
      | Torque_Nm_Motor = TorqueActualValue/1000 * ratedTorque
      | ratedTorque = ratedCurrent * motorConstant
  TorqueActualValue : Inport
  Data Type Conversion6 : DataTypeConversion  OutDataTypeStr=double
  GearboxRatio : Constant  Value=ActuatorStruct.GearboxRatio
  MagicConstant : Constant  Value=1/1000
  MotorConstant : Constant  Value=ActuatorStruct.Motor.MotorConstant_Nm_A
  Product : Product  Inputs=5
  RatedCurrent : Constant  Value=ActuatorStruct.Motor.RatedCurrent_A
  MotorTorque_Nm : Outport  VectorParamsAs1DForOutWhenUnconnected=off
  wires:
  RatedCurrent/1 -> Product/3
  MotorConstant/1 -> Product/4
  GearboxRatio/1 -> Product/5
  MagicConstant/1 -> Product/2
  TorqueActualValue/1 -> Data Type Conversion6/1
  Product/1 -> MotorTorque_Nm/1
  Data Type Conversion6/1 -> Product/1

== system WEankle_controllerMaarten_2018/FromActuators/RA/ToMotorVelocity_rad_s ==
  note: This block outputs the velocity of the axis connected to the motor, AFTER the gearbox (so it has the same order of magnitude as, and directly comparable to JointVelocity_rad_s).
  note: VelocityActualValue (v_IU for short) is in mrev/s (milli-revolutions per second)
      |
      | We want the motor velocity converted to the output shaft:
      |
      |
      | MotorVelocity_rad_s_outputshaft = MotorVelocity_rad_s_motorshaft / gearboxRatio
      | MotorVelocity_rad_s_motorshaft = v_IU / 1000 * 2 * pi
      |
      | (no sample time inolved in the conversion here; the v_IU is already in per-second)
  VelocityActualValue : Inport
  Data Type Conversion6 : DataTypeConversion  OutDataTypeStr=double
  OneOverGearboxRatio : Constant  Value=1/ActuatorStruct.GearboxRatio
  Product : Product  Inputs=***
  TwoPiOverThousand : Constant  Value=2*pi / 1000
  MotorVelocity_rad_s : Outport  VectorParamsAs1DForOutWhenUnconnected=off
  wires:
  TwoPiOverThousand/1 -> Product/2
  OneOverGearboxRatio/1 -> Product/3
  Data Type Conversion6/1 -> Product/1
  Product/1 -> MotorVelocity_rad_s/1
  VelocityActualValue/1 -> Data Type Conversion6/1

== system WEankle_controllerMaarten_2018/Ankle Controller/COMverror and perturbation/COMvError/Data lost detection ==
  note: Assuming no data lost
  Input signal : Inport
  ErrorIn : Inport  Port=2
  Delay : Delay  DelayLength=1
  Delay1 : Delay  DelayLength=1
  Gain1 : Gain  Gain=0
  Gain2 : Gain  Gain=100
  MATLAB Function1 : MATLAB Function  TreatAsAtomicUnit=on
  MATLAB Function2 : MATLAB Function  TreatAsAtomicUnit=on
  New error : Outport  VectorParamsAs1DForOutWhenUnconnected=off
  DataLost : Outport  Port=2  VectorParamsAs1DForOutWhenUnconnected=off
  avoid : Outport  Port=3  VectorParamsAs1DForOutWhenUnconnected=off
  wires:
  MATLAB Function2/2(avoid) -> avoid/1
  ErrorIn/1 -> MATLAB Function2/3(ErrorIn)
  Delay/1 -> MATLAB Function1/2(u_1)
  MATLAB Function2/1(ErrorOut) -> New error/1  "New error"
  Delay1/1 -> MATLAB Function2/2(DataLost_1)
  Input signal/1 -> MATLAB Function1/1(u), Delay/1
  MATLAB Function1/1(y) -> Gain1/1
  Gain2/1 -> DataLost/1  "DataLost"
  Gain1/1 -> Delay1/1, MATLAB Function2/1(DataLost), Gain2/1  "DataLost"

== system WEankle_controllerMaarten_2018/Ankle Controller/COMverror and perturbation/COMvError/PertDetection ==
  PertFromError : Inport
  PertFromInputSignal : Inport  Port=2
  avoid : Inport  Port=3
  Delay : Delay  DelayLength=1
  Detect Increase : simulink/Logic and Bit Operations/Detect Increase  vinit=0  OutDataTypeStr=boolean
  MATLAB Function1 : MATLAB Function  TreatAsAtomicUnit=on
  MATLAB Function2 : MATLAB Function  TreatAsAtomicUnit=on
  PertDetect : Outport  VectorParamsAs1DForOutWhenUnconnected=off
  wires:
  Detect Increase/1 -> MATLAB Function1/4(StartPertFromError)
  Delay/1 -> MATLAB Function2/2(Pert_1)
  MATLAB Function1/1(PertDetect) -> Delay/1, MATLAB Function2/1(Pert)
  PertFromInputSignal/1 -> MATLAB Function1/2(PertFromInput)
  MATLAB Function2/1(PertDetect) -> PertDetect/1
  PertFromError/1 -> MATLAB Function1/1(PertFromError), Detect Increase/1
  avoid/1 -> MATLAB Function1/3(avoid)

== system WEankle_controllerMaarten_2018/Ankle Controller/COMverror and perturbation/COMvError/Signal learner ==
  note: To convert pos to vel
  note: Excluding for the average those steps where a perturbation happened.
      | The threshold to calculate which steps where perturbed is taken as the
      | mean of maximums in previous steps. Avoiding DataLost and false Triggers
  Signaltime : Inport
  trigger : Inport  Port=2
  xPosCOM : Inport  Port=3
  Constant : Constant  Value=5
  Constant1 : Constant  Value=1.5
  Discrete Derivative1 : simulink/Discrete/Discrete Derivative  gainval=1.0  ICPrevScaledInput=0.0  OutMin=[]  OutMax=[]  OutDataType=fixdt(1, 16)  OutScaling=2^-10  DoSatur=off
  Lowpass Filter2 : dspfdesign/Lowpass Filter  FilterType=IIR  DesignForMinimumOrder=on  FilterOrder=50  PassbandFrequency=5  StopbandFrequency=50  PassbandRipple=0.1  StopbandAttenuation=40  InheritSampleRate=off  SampleRate=1000  SimulateUsing=Interpreted execution  roundingMode=Floor  coeffsDataTypeStr=fixdt(1,16)
  MATLAB Function : MATLAB Function  TreatAsAtomicUnit=on
  MATLAB Function1 : MATLAB Function  Commented=on  TreatAsAtomicUnit=on
  Rate Transition : RateTransition
  Sum : Sum  Inputs=|+-
  original : Outport  VectorParamsAs1DForOutWhenUnconnected=off
  error : Outport  Port=2  VectorParamsAs1DForOutWhenUnconnected=off
  Input filtered : Outport  Port=3  VectorParamsAs1DForOutWhenUnconnected=off
  learned : Outport  Port=4  VectorParamsAs1DForOutWhenUnconnected=off
  Perturbation detected FromInput : Outport  Port=5  VectorParamsAs1DForOutWhenUnconnected=off
  ShutDown : Outport  Port=6  VectorParamsAs1DForOutWhenUnconnected=off
  tag scope: m=global, n=global, n_strides=global, stride_duration=global
  wires:
  MATLAB Function/7(ShutDown) -> ShutDown/1
  [DataLost] -> MATLAB Function/7(DataLost)  "DataLost"
  Constant1/1 -> MATLAB Function/6(threshPert)
  MATLAB Function/6(perturbation) -> Perturbation detected FromInput/1
  trigger/1 -> MATLAB Function/3(trigger)
  Sum/1 -> error/1  "error"
  Signaltime/1 -> MATLAB Function/2(t)
  MATLAB Function/5(output_duration_) -> [stride_duration]  "stride_duration"
  Constant/1 -> MATLAB Function/5(n_rep)
  MATLAB Function/4(m_) -> [m]  "m"
  MATLAB Function/1(signal_learned) -> Sum/2, learned/1  "learned"
  MATLAB Function/2(n_strides_) -> [n_strides]  "n_strides"
  MATLAB Function/3(n_) -> [n]  "n"
  Lowpass Filter2/1 -> Sum/1, Input filtered/1, MATLAB Function/4(signal)  "prev"
  xPosCOM/1 -> Discrete Derivative1/1  "original"
  Discrete Derivative1/1 -> Rate Transition/1  "original"
  Rate Transition/1 -> original/1, Lowpass Filter2/1
  [Reset] -> MATLAB Function/1(reset)

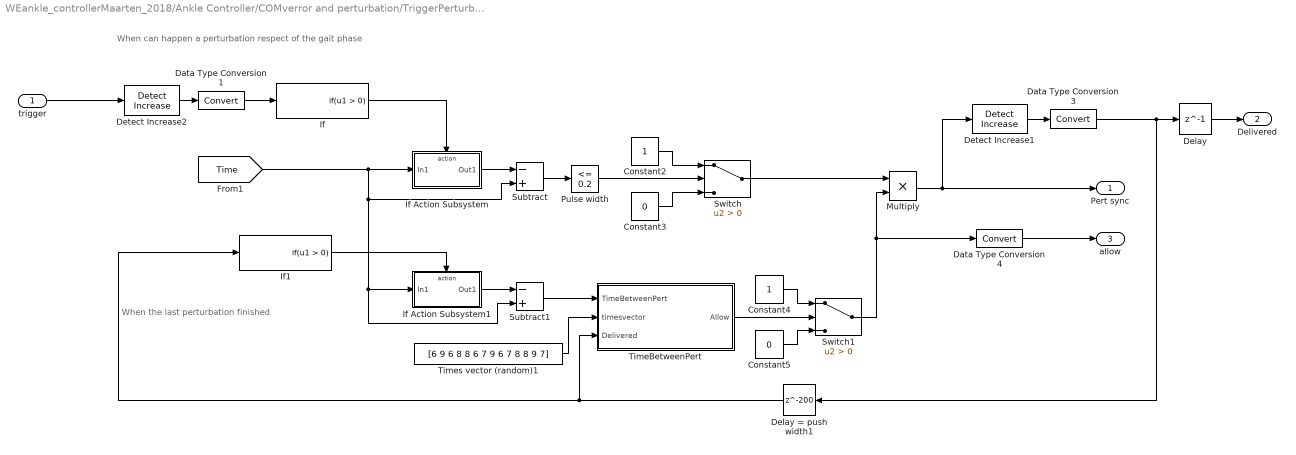
== system WEankle_controllerMaarten_2018/Ankle Controller/COMverror and perturbation/TriggerPerturbation/Perturbation sync gait phase1 ==
  note: When the last perturbation finished
  note: When can happen a perturbation respect of the gait phase
  trigger : Inport
  Constant2 : Constant
  Constant3 : Constant  Value=0
  Constant4 : Constant
  Constant5 : Constant  Value=0
  Data Type Conversion1 : DataTypeConversion
  Data Type Conversion3 : DataTypeConversion
  Data Type Conversion4 : DataTypeConversion
  Delay : Delay  DelayLength=1
  Delay = push width1 : Delay  DelayLength=200  InitialCondition=0
  Detect Increase1 : simulink/Logic and Bit Operations/Detect Increase  vinit=0  OutDataTypeStr=boolean
  Detect Increase2 : simulink/Logic and Bit Operations/Detect Increase  vinit=0  OutDataTypeStr=boolean
  If : If  ShowElse=off
  If Action Subsystem : Subsystem  TreatAsAtomicUnit=on
  If Action Subsystem1 : Subsystem  TreatAsAtomicUnit=on
  If1 : If  ShowElse=off
  Multiply : Product
  Pulse width : simulink/Logic and Bit Operations/Compare To Constant  relop=<=  const=0.2  OutDataTypeStr=boolean
  Subtract : Sum  Inputs=-+
  Subtract1 : Sum  Inputs=-+
  Switch : Switch  Criteria=u2 > Threshold
  Switch1 : Switch  Criteria=u2 > Threshold
  TimeBetweenPert : MATLAB Function  TreatAsAtomicUnit=on
  Times vector (random)1 : Constant  Value=[6 9 6 8 8 6 7 9 6 7 8 8 9 7]
  Pert sync : Outport  VectorParamsAs1DForOutWhenUnconnected=off
  Delivered : Outport  Port=2  VectorParamsAs1DForOutWhenUnconnected=off
  allow : Outport  Port=3  VectorParamsAs1DForOutWhenUnconnected=off
  wires:
  Times vector (random)1/1 -> TimeBetweenPert/2(timesvector)
  Subtract1/1 -> TimeBetweenPert/1(TimeBetweenPert)
  TimeBetweenPert/1(Allow) -> Switch1/2
  Data Type Conversion4/1 -> allow/1
  Delay/1 -> Delivered/1
  Data Type Conversion3/1 -> Delay/1, Delay = push width1/1
  Delay = push width1/1 -> If1/1, TimeBetweenPert/3(Delivered)
  If1/1 -> If Action Subsystem1/Action
  Constant3/1 -> Switch/3
  If/1 -> If Action Subsystem/Action
  Constant2/1 -> Switch/1
  [Time] -> Subtract1/2, If Action Subsystem1/1(In1), Subtract/2, If Action Subsystem/1(In1)
  Constant5/1 -> Switch1/3
  Pulse width/1 -> Switch/2
  Multiply/1 -> Detect Increase1/1, Pert sync/1
  If Action Subsystem/1(Out1) -> Subtract/1
  If Action Subsystem1/1(Out1) -> Subtract1/1
  trigger/1 -> Detect Increase2/1
  Subtract/1 -> Pulse width/1
  Switch/1 -> Multiply/1
  Switch1/1 -> Multiply/2, Data Type Conversion4/1
  Detect Increase2/1 -> Data Type Conversion1/1
  Data Type Conversion1/1 -> If/1
  Constant4/1 -> Switch1/1
  Detect Increase1/1 -> Data Type Conversion3/1

== system WEankle_controllerMaarten_2018/Ankle Controller/Gait Phase detection/COP detection (treadmill)/Get_COPL ==
  note: COPx
  note: COPy
  grf : Inport
  Enable : EnablePort  StatesWhenEnabling=reset
  Demux1 : Demux  Outputs=3
  Divide : Product  Inputs=*/
  Divide1 : Product  Inputs=*/
  Gain : Gain  Gain=-1
  LEFT Mx My Fz : Selector  InputPortWidth=6  IndexOptions=Index vector (dialog)  Indices=[4 5 3]  OutputSizes=1
  Mux : Mux  Inputs=2
  COPL : Outport  OutputWhenDisabled=reset  InitialOutput=0  VectorParamsAs1DForOutWhenUnconnected=off
  wires:
  grf/1 -> LEFT Mx My Fz/1
  LEFT Mx My Fz/1 -> Demux1/1
  Demux1/2 -> Gain/1  "My"
  Gain/1 -> Divide/1
  Demux1/3 -> Divide1/2, Divide/2  "Fz"
  Demux1/1 -> Divide1/1  "Mx"
  Divide/1 -> Mux/1
  Divide1/1 -> Mux/2
  Mux/1 -> COPL/1

== system WEankle_controllerMaarten_2018/Ankle Controller/Gait Phase detection/COP detection (treadmill)/Get_COPR ==
  note: COPx
  note: COPy
  grf : Inport
  Enable : EnablePort  StatesWhenEnabling=reset
  Demux1 : Demux  Outputs=3
  Divide : Product  Inputs=*/
  Divide1 : Product  Inputs=*/
  Gain : Gain  Gain=-1
  Mux : Mux  Inputs=2
  RIGHT Mx My Fz : Selector  InputPortWidth=6  IndexOptions=Index vector (dialog)  Indices=[4 5 3]  OutputSizes=1
  COPR : Outport  OutputWhenDisabled=reset  InitialOutput=0  VectorParamsAs1DForOutWhenUnconnected=off
  wires:
  grf/1 -> RIGHT Mx My Fz/1
  RIGHT Mx My Fz/1 -> Demux1/1
  Demux1/2 -> Gain/1  "My"
  Gain/1 -> Divide/1
  Demux1/3 -> Divide1/2, Divide/2  "Fz"
  Demux1/1 -> Divide1/1  "Mx"
  Divide/1 -> Mux/1
  Divide1/1 -> Mux/2
  Mux/1 -> COPR/1

== system WEankle_controllerMaarten_2018/FromActuators/RA/ToJointAngle_rad/FilterFourthOrder ==
  note: Set Omega to 0 to disable filter
  In : Inport
  Omega : Inport  Port=2
  Filter1 : MATLAB Function  TreatAsAtomicUnit=on  mask{sampleTime=sampleTime}
      mask prompts: sampleTime "Sample Time"
  Filter2 : MATLAB Function  TreatAsAtomicUnit=on  mask{sampleTime=sampleTime}
      mask prompts: sampleTime "Sample Time"
  Out : Outport  VectorParamsAs1DForOutWhenUnconnected=off
  wires:
  Filter1/1(y) -> Filter2/1(x)
  Omega/1 -> Filter2/2(OmegaFilter), Filter1/2(OmegaFilter)
  In/1 -> Filter1/1(x)
  Filter2/1(y) -> Out/1
